simulink model "fig9_22"  (Simulink 7.0)
settings: Solver=ode45  SolverMode=SingleTasking  StartTime=0.0  StopTime=10.0  RelTol=1e-3  AbsTol=1e-6
undefined symbols (not defined in the file or in its folder): ka
settings Model: Creator=abbas  LastModifiedBy=abbas  ExtModeTrigMode=oneshot  ExtModeArmWhenConnect=off
settings DataIOCC: LimitDataPoints=off
settings OptimizationCC: BlockReduction=off  BooleanDataType=off  InlineInvariantSignals=on
settings DebuggingCC: SaveWithParameterizedLinksMsg=none  SignalResolutionControl=TryResolveAllWithWarning  SolverPrmCheckMsg=none  MultiTaskDSMMsg=warning  MultiTaskCondExecSysMsg=none  StrictBusMsg=None
settings HardwareCC: TargetUnknown=on
settings RTWCC: IncludeERTFirstTime=on
settings GRTTargetCC: TargetFcnLib=ansi_tfl_tmw.mat  ModelReferenceCompliant=off  CompOptLevelCompliant=off  MatFileLogging=off

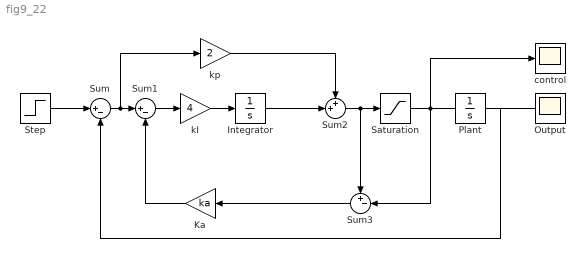
== system fig9_22 ==
  Integrator : Integrator
  Ka : Gain  Orientation=left  Gain=ka  ParameterDataType=sfix(16)  ParameterScaling=2^0  OutDataType=sfix(16)  OutScaling=2^0  SaturateOnIntegerOverflow=on
  Output : Scope
      settings: TickLabels=on  SaveName=yantib  DataFormat=Array
  Plant : Integrator
  Saturation : Saturate  UpperLimit=1.0  LowerLimit=-1.0
  Step : Step  Time=.2  SampleTime=0.01
  Sum : Sum  Inputs=|+-  OutDataType=sfix(16)  OutScaling=2^0  SaturateOnIntegerOverflow=on  InputSameDT=on
  Sum1 : Sum  Inputs=|+-  OutDataType=sfix(16)  OutScaling=2^0  SaturateOnIntegerOverflow=on  InputSameDT=on
  Sum2 : Sum  Inputs=++|  OutDataType=sfix(16)  OutScaling=2^0  SaturateOnIntegerOverflow=on  InputSameDT=on
  Sum3 : Sum  Orientation=left  Inputs=+-|  OutDataType=sfix(16)  OutScaling=2^0  InputSameDT=on
  control : Scope
      settings: TickLabels=on  SaveName=uantib  DataFormat=Array
  kI : Gain  Gain=4  ParameterDataType=sfix(16)  ParameterScaling=2^0  OutDataType=sfix(16)  OutScaling=2^0
  kp : Gain  Gain=2  ParameterDataType=sfix(16)  ParameterScaling=2^0  OutDataType=sfix(16)  OutScaling=2^0
  wires:
  kI/1 -> Integrator/1
  Plant/1 -> Output/1, Sum/2
  Saturation/1 -> Sum3/2, Plant/1, control/1
  Sum1/1 -> kI/1
  Sum3/1 -> Ka/1
  Step/1 -> Sum/1
  Ka/1 -> Sum1/2
  Sum2/1 -> Saturation/1, Sum3/1
  Integrator/1 -> Sum2/2
  kp/1 -> Sum2/1
  Sum/1 -> Sum1/1, kp/1
